simulink model "Discrete_Transfer_Fcn_Test_Model"  (R2019b)
settings: Solver=VariableStepAuto  StartTime=0.0  StopTime=testtime  RelTol=1e-3
InitFcn:
  | Discrete_Transfer_Fcn_Test_Parameters
StopFcn:
  | Verify_Discrete_Transfer_Fcn_Test_Filter
values from neighbouring files (symbols this model uses):
  c1LPihc = ( C - TWOPI*Fcihc ) / ( C + TWOPI*Fcihc )    (= 0.671752219322)    [Discrete_Transfer_Fcn_Test_Parameters.m]
  c2LPihc = TWOPI*Fcihc / (TWOPI*Fcihc + C)    (= 0.164123890339)    [Discrete_Transfer_Fcn_Test_Parameters.m]
  Fs = 48e3    (= 48000)    [Discrete_Transfer_Fcn_Test_Parameters.m]
  gainihc = 1.0    (= 1)    [Discrete_Transfer_Fcn_Test_Parameters.m]
undefined symbols (not defined in the file or in its folder): dfilt
libraries: dsparch4 x2, dspsrcs4 x1
settings Model: Creator=mblun  LastModifiedBy=cb50701
settings OptimizationCC: BlockReduction=off  ConditionallyExecuteInputs=off  DefaultParameterBehavior=Inlined
settings DebuggingCC: AlgebraicLoopMsg=error
settings HardwareCC: ProdBitPerPointer=32  ProdBitPerSizeT=32  ProdBitPerPtrDiffT=32  ProdLargestAtomicFloat=None  ProdIntDivRoundTo=Undefined  ProdEndianess=Unspecified  ProdWordSize=32  ProdHWDeviceType=ASIC/FPGA->ASIC/FPGA  TargetBitPerLong=64  TargetBitPerPointer=64  TargetBitPerSizeT=64  TargetBitPerPtrDiffT=64  TargetLongLongMode=on  TargetIntDivRoundTo=Zero  TargetEndianess=LittleEndian  TargetWordSize=64  TargetHWDeviceType=Custom Processor->MATLAB Host Computer  ProdEqTarget=off
settings SFSimCC: CustomCodeUndefinedFunction=UseInterfaceOnly

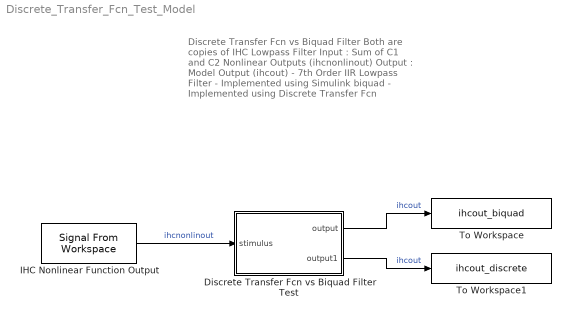
== system Discrete_Transfer_Fcn_Test_Model ==
  note: Discrete Transfer Fcn vs Biquad Filter
      | Both are copies of IHC Lowpass Filter
      |
      | Input : Sum of C1 and C2 Nonlinear Outputs (ihcnonlinout)
      |
      | Output : Model Output (ihcout)
      |
      | - 7th Order IIR Lowpass Filter
      |
      | - Implemented using Simulink biquad
      |
      | - Implemented using Discrete Transfer Fcn
  Discrete Transfer Fcn vs Biquad Filter Test : Subsystem
  IHC Nonlinear Function Output : dspsrcs4/Signal From Workspace  X=RxSignal  Ts=1/Fs  nsamps=1  OutputAfterFinalValue=Setting to zero  ignoreOrWarnInputAndFrameLengths=off  OutputFrames=off
  To Workspace : ToWorkspace  VariableName=ihcout_biquad  SampleTime=-1
      settings: Save2DSignal=2-D array (concatenate along first dimension)
  To Workspace1 : ToWorkspace  VariableName=ihcout_discrete  SampleTime=-1
      settings: Save2DSignal=2-D array (concatenate along first dimension)
  wires:
  Discrete Transfer Fcn vs Biquad Filter Test/1(output) -> To Workspace/1  "ihcout"
  IHC Nonlinear Function Output/1 -> Discrete Transfer Fcn vs Biquad Filter Test/1(stimulus)  "ihcnonlinout"
  Discrete Transfer Fcn vs Biquad Filter Test/2(output1) -> To Workspace1/1  "ihcout"

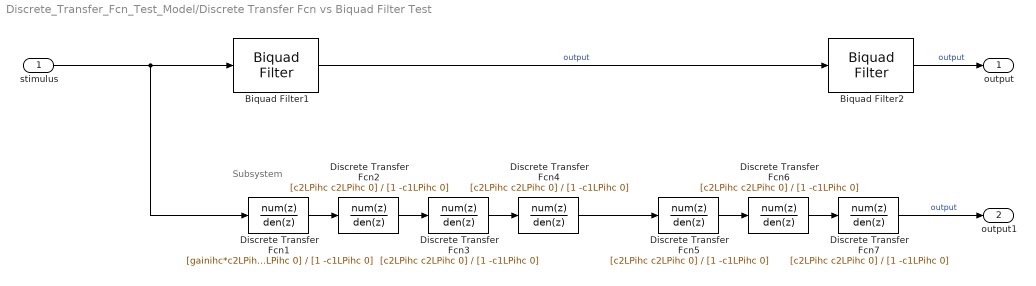
== system Discrete_Transfer_Fcn_Test_Model/Discrete Transfer Fcn vs Biquad Filter Test ==
  note: Subsystem
  stimulus : Inport
  Biquad Filter1 : dsparch4/Biquad Filter  FilterSource=Dialog parameters  CoeffSource=Specify via dialog  FilterObject=dfilt.df2tsos([1 0.3 0.4],[1 0.1 0.2])  IIRFiltStruct=Direct form II transposed  BiQuadCoeffs=[gainihc*c2LPihc gainihc*c2LPihc 0 1 -c1LPihc 0; c2LPihc c2LPihc 0 1 -c1LPihc 0; c2LPihc c2LPihc 0 1 -c1LPihc 0;c2LPihc c2LPihc 0 1 -c1LPihc 0]  ScaleValues=1  IC=0  ICnum=0  ICden=0  a0Flag=Warning  optimizeScaleValues=on  ScaleValueMode=Specify via input port (g)  roundingMode=Floor  overflowMode=on  scaleValueFracLength=14  denProdOutputFracLength=30  denAccumFracLength=30  secondMemoryFracLength=15
      settings: SourceProductName=DSP System Toolbox
  Biquad Filter2 : dsparch4/Biquad Filter  FilterSource=Dialog parameters  CoeffSource=Specify via dialog  FilterObject=dfilt.df2tsos([1 0.3 0.4],[1 0.1 0.2])  IIRFiltStruct=Direct form II transposed  BiQuadCoeffs=[c2LPihc c2LPihc 0 1 -c1LPihc 0; c2LPihc c2LPihc 0 1 -c1LPihc 0; c2LPihc c2LPihc 0 1 -c1LPihc 0]  ScaleValues=1  IC=0  ICnum=0  ICden=0  a0Flag=Warning  optimizeScaleValues=on  ScaleValueMode=Specify via input port (g)  roundingMode=Floor  overflowMode=on  scaleValueFracLength=14  denProdOutputFracLength=30  denAccumFracLength=30  secondMemoryFracLength=15
      settings: SourceProductName=DSP System Toolbox
  Discrete Transfer Fcn1 : DiscreteTransferFcn  Numerator=[gainihc*c2LPihc gainihc*c2LPihc 0]  Denominator=[1 -c1LPihc 0]
  Discrete Transfer Fcn{2..7} (6 alike) : DiscreteTransferFcn  Numerator=[c2LPihc c2LPihc 0]  Denominator=[1 -c1LPihc 0]
  output : Outport  VectorParamsAs1DForOutWhenUnconnected=off
  output1 : Outport  Port=2  VectorParamsAs1DForOutWhenUnconnected=off
  wires:
  Biquad Filter1/1 -> Biquad Filter2/1  "output"
  Biquad Filter2/1 -> output/1  "output"
  Discrete Transfer Fcn6/1 -> Discrete Transfer Fcn7/1
  Discrete Transfer Fcn7/1 -> output1/1  "output"
  Discrete Transfer Fcn4/1 -> Discrete Transfer Fcn5/1
  stimulus/1 -> Discrete Transfer Fcn1/1, Biquad Filter1/1
  Discrete Transfer Fcn5/1 -> Discrete Transfer Fcn6/1
  Discrete Transfer Fcn3/1 -> Discrete Transfer Fcn4/1
  Discrete Transfer Fcn2/1 -> Discrete Transfer Fcn3/1
  Discrete Transfer Fcn1/1 -> Discrete Transfer Fcn2/1
